simulink library "mantaFSHiLvl_cl"  (R2020a)
settings: Solver=VariableStepAuto  StartTime=0.0  StopTime=10.0  RelTol=1e-3
undefined symbols (not defined in the file or in its folder): fltCtrl, HILVLCONTROLLER, hiLvlCtrl, initializeBussesFromBlock
libraries: simulink x5, vectorMagnitude_ul x3, stopwatch_ul x1, pathFollowingControllerManta_cl x1
settings Model: Creator=mcobb  LastModifiedBy=JohnJr
settings DataIOCC: ReturnWorkspaceOutputs=off
settings DebuggingCC: ArithmeticOperatorsInVariantConditions=warning
settings SFSimCC: CustomCodeUndefinedFunction=UseInterfaceOnly

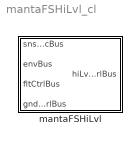
== system mantaFSHiLvl_cl ==
  mantaFSHiLvl : Subsystem  LoadFcn=initializeBussesFromBlock(gcb)  InitFcn=initializeBussesFromBlock(gcb)  StartFcn=initializeBussesFromBlock(gcb)  VariantControl=strcmpi(HILVLCONTROLLER,'mantaFSHiLvl')  mask{hiLvlCtrl=hiLvlCtrl}
      mask prompts: hiLvlCtrl "Hi-level controller"

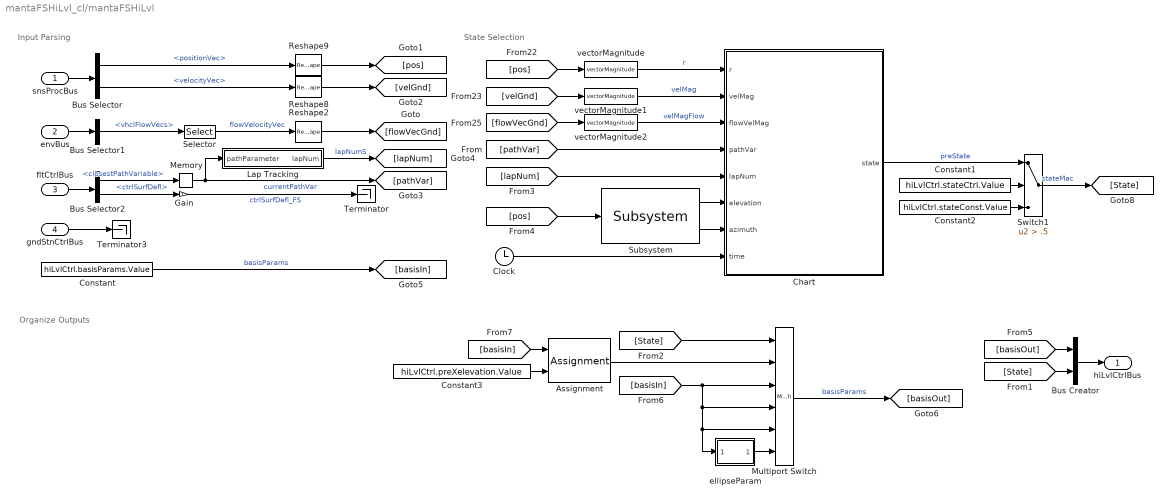
== system mantaFSHiLvl_cl/mantaFSHiLvl ==
  note: Organize Outputs
  note: Input Parsing
  note: State Selection
  snsProcBus : Inport  OutDataTypeStr=Bus: sensorsProcessingBus
  envBus : Inport  Port=2  OutDataTypeStr=Bus: envBus
  fltCtrlBus : Inport  Port=3  OutDataTypeStr=Bus: fltCtrlBus
  gndStnCtrlBus : Inport  Port=4  OutDataTypeStr=Bus: gndStnCtrlBus
  Assignment : Assignment  DiagnosticForDimensions=Warning  IndexOptions=Index vector (dialog)  Indices=3  OutputSizes=1
  Bus Creator : BusCreator  Inputs=2  OutDataTypeStr=Bus: hiLvlCtrlBus
  Bus Selector : BusSelector  OutputSignals=positionVec,velocityVec
  Bus Selector1 : BusSelector  OutputSignals=vhclFlowVecs
  Bus Selector2 : BusSelector  OutputSignals=closestPathVariable,ctrlSurfDefl
  Chart : Stateflow chart  TreatAsAtomicUnit=on  mask{nonXGain=fltCtrl.nonXCurrentSpoolInGain.Value, maxR=fltCtrl.maxTL.Value}
      mask prompts: nonXGain "non-xcurrent spool speed gain"; maxR "max kite position magnitude (r)"
  Clock : Clock
  Constant : Constant  Value=hiLvlCtrl.basisParams.Value
  Constant1 : Constant  Value=hiLvlCtrl.stateCtrl.Value
  Constant2 : Constant  Value=hiLvlCtrl.stateConst.Value
  Constant3 : Constant  Value=hiLvlCtrl.preXelevation.Value
  Gain : Gain
  Lap Tracking : Subsystem
  Memory : Memory
  Multiport Switch : MultiPortSwitch  Inputs=5
  Reshape2 : Reshape  OutputDimensionality=Column vector (2-D)
  Reshape8 : Reshape  OutputDimensionality=Column vector (2-D)
  Reshape9 : Reshape  OutputDimensionality=Column vector (2-D)
  Selector : Selector  NumberOfDimensions=2  InputPortWidth=3  IndexOptions=Select all,Index vector (dialog)  Indices=[1 3],5  OutputSizes=1,1
  Subsystem : pathFollowingControllerManta_cl/pathFollowingControllerManta/Subsystem  SystemSampleTime=-1  Latency=0  AutoFrameSizeCalculation=off
  Switch1 : Switch  Criteria=u2 > Threshold  Threshold=.5
  Terminator : Terminator
  Terminator3 : Terminator
  ellipseParam : Subsystem
  vectorMagnitude : vectorMagnitude_ul/vectorMagnitude  SystemSampleTime=-1  Latency=0  AutoFrameSizeCalculation=off
  vectorMagnitude1 : vectorMagnitude_ul/vectorMagnitude  SystemSampleTime=-1  Latency=0  AutoFrameSizeCalculation=off
  vectorMagnitude2 : vectorMagnitude_ul/vectorMagnitude  SystemSampleTime=-1  Latency=0  AutoFrameSizeCalculation=off
  hiLvlCtrlBus : Outport  OutDataTypeStr=Bus: hiLvlCtrlBus  VectorParamsAs1DForOutWhenUnconnected=off
  wires:
  gndStnCtrlBus/1 -> Terminator3/1
  Bus Creator/1 -> hiLvlCtrlBus/1
  Reshape9/1 -> [pos]
  snsProcBus/1 -> Bus Selector/1
  Reshape8/1 -> [velGnd]
  Bus Selector/2 -> Reshape8/1  "<velocityVec>"
  Bus Selector/1 -> Reshape9/1  "<positionVec>"
  Bus Selector1/1 -> Selector/1  "<vhclFlowVecs>"
  Reshape2/1 -> [flowVecGnd]
  envBus/1 -> Bus Selector1/1
  Selector/1 -> Reshape2/1  "flowVelocityVec"
  [State] -> Bus Creator/2
  [pos] -> vectorMagnitude/1
  [velGnd] -> vectorMagnitude1/1
  [flowVecGnd] -> vectorMagnitude2/1
  vectorMagnitude/1 -> Chart/1(r)  "r"
  vectorMagnitude1/1 -> Chart/2(velMag)  "velMag"
  vectorMagnitude2/1 -> Chart/3(flowVelMag)  "velMagFlow"
  fltCtrlBus/1 -> Bus Selector2/1
  Bus Selector2/1 -> Memory/1  "<closestPathVariable>"
  Memory/1 -> [pathVar], Lap Tracking/1(pathParameter)  "currentPathVar"
  Lap Tracking/1(lapNum) -> [lapNum]  "lapNumS"
  [pathVar] -> Chart/4(pathVar)
  [lapNum] -> Chart/5(lapNum)
  Subsystem/1 -> Chart/6(elevation)
  Subsystem/2 -> Chart/7(azimuth)
  [pos] -> Subsystem/1
  Clock/1 -> Chart/8(time)
  Switch1/1 -> [State]  "stateMac"
  Chart/1(state) -> Switch1/1  "preState"
  Constant1/1 -> Switch1/2
  Constant2/1 -> Switch1/3
  Constant/1 -> [basisIn]  "basisParams"
  [State] -> Multiport Switch/1
  [basisIn] -> Multiport Switch/3, Multiport Switch/4, Multiport Switch/5, ellipseParam/1(In1)
  ellipseParam/1(Out1) -> Multiport Switch/6
  Multiport Switch/1 -> [basisOut]  "basisParams"
  [basisOut] -> Bus Creator/1
  [basisIn] -> Assignment/1
  Assignment/1 -> Multiport Switch/2
  Constant3/1 -> Assignment/2
  Bus Selector2/2 -> Gain/1  "<ctrlSurfDefl>"
  Gain/1 -> Terminator/1  "ctrlSurfDefl_FS"

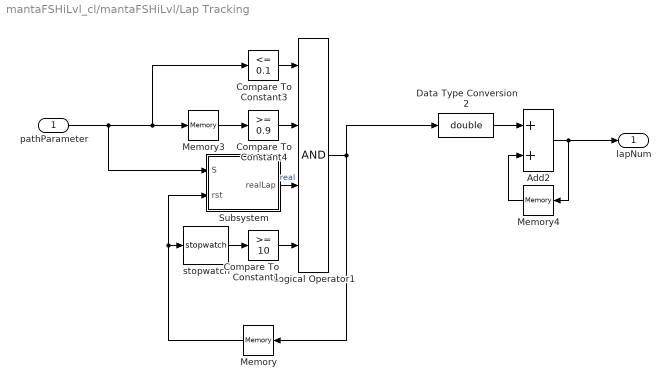
== system mantaFSHiLvl_cl/mantaFSHiLvl/Lap Tracking ==
  pathParameter : Inport
  Add2 : Sum
  Compare To Constant1 : simulink/Logic and Bit Operations/Compare To Constant  relop=>=  const=10  OutDataTypeStr=boolean
  Compare To Constant3 : simulink/Logic and Bit Operations/Compare To Constant  relop=<=  const=0.1  OutDataTypeStr=boolean
  Compare To Constant4 : simulink/Logic and Bit Operations/Compare To Constant  relop=>=  const=0.9  OutDataTypeStr=boolean
  Data Type Conversion2 : DataTypeConversion  OutDataTypeStr=double
  Logical Operator1 : Logic  Inputs=4  AllPortsSameDT=off  OutDataTypeStr=boolean
  Memory : Memory  InitialCondition=false
  Memory3 : Memory
  Memory4 : Memory
  Subsystem : Subsystem
  stopwatch : stopwatch_ul/stopwatch  SystemSampleTime=-1  Latency=0  AutoFrameSizeCalculation=off
  lapNum : Outport  VectorParamsAs1DForOutWhenUnconnected=off
  wires:
  Subsystem/1(realLap) -> Logical Operator1/3  "real"
  Compare To Constant1/1 -> Logical Operator1/4
  Memory/1 -> stopwatch/1, Subsystem/2(rst)
  stopwatch/1 -> Compare To Constant1/1
  pathParameter/1 -> Memory3/1, Compare To Constant3/1, Subsystem/1(S)
  Compare To Constant4/1 -> Logical Operator1/2
  Add2/1 -> Memory4/1, lapNum/1
  Memory4/1 -> Add2/2
  Logical Operator1/1 -> Memory/1, Data Type Conversion2/1
  Data Type Conversion2/1 -> Add2/1
  Memory3/1 -> Compare To Constant4/1
  Compare To Constant3/1 -> Logical Operator1/1

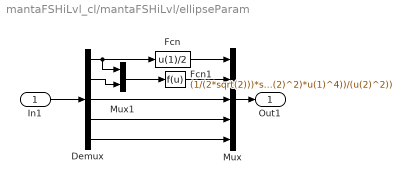
== system mantaFSHiLvl_cl/mantaFSHiLvl/ellipseParam ==
  In1 : Inport
  Demux : Demux  Outputs=5
  Fcn : Fcn  Expr=u(1)/2
  Fcn1 : Fcn  Expr=(1/(2*sqrt(2)))*sqrt(-u(1)^2+sqrt((u(2)^2*(4+u(2)^2)*u(1)^4))/(u(2)^2))
  Mux : Mux  Inputs=5
  Mux1 : Mux  Inputs=2
  Out1 : Outport
  wires:
  In1/1 -> Demux/1
  Mux1/1 -> Fcn1/1
  Demux/4 -> Mux/4
  Mux/1 -> Out1/1
  Fcn1/1 -> Mux/2
  Demux/2 -> Mux1/2
  Demux/1 -> Mux1/1, Fcn/1
  Fcn/1 -> Mux/1
  Demux/5 -> Mux/5
  Demux/3 -> Mux/3

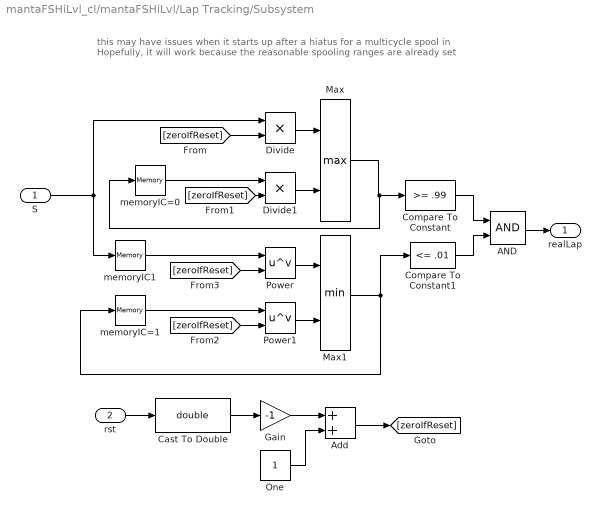
== system mantaFSHiLvl_cl/mantaFSHiLvl/Lap Tracking/Subsystem ==
  note: this may have issues when it starts up after a hiatus for a multicycle spool in
      | Hopefully, it will work because the reasonable spooling ranges are already set
  S : Inport
  rst : Inport  Port=2
  AND : Logic  AllPortsSameDT=off  OutDataTypeStr=boolean
  Add : Sum
  Cast To Double : DataTypeConversion  OutDataTypeStr=double
  Compare To Constant : simulink/Logic and Bit Operations/Compare To Constant  relop=>=  const=.99  OutDataTypeStr=boolean
  Compare To Constant1 : simulink/Logic and Bit Operations/Compare To Constant  relop=<=  const=.01  OutDataTypeStr=boolean
  Divide : Product  Inputs=**
  Divide1 : Product  Inputs=**
  Gain : Gain  Gain=-1
  Max : MinMax  Function=max  Inputs=2
  Max1 : MinMax  Inputs=2
  One : Constant  OutDataTypeStr=Inherit: Inherit via back propagation
  Power : Math  Operator=pow  SaturateOnIntegerOverflow=on
  Power1 : Math  Operator=pow  SaturateOnIntegerOverflow=on
  memoryIC1 : Memory  InitialCondition=1
  memoryIC=0 : Memory
  memoryIC=1 : Memory  InitialCondition=1
  realLap : Outport
  wires:
  memoryIC1/1 -> Power/1
  memoryIC=1/1 -> Power1/1
  [zeroIfReset] -> Power1/2
  memoryIC=0/1 -> Divide1/1
  Divide1/1 -> Max/2
  [zeroIfReset] -> Divide1/2
  [zeroIfReset] -> Power/2
  [zeroIfReset] -> Divide/2
  AND/1 -> realLap/1
  Compare To Constant1/1 -> AND/2
  Compare To Constant/1 -> AND/1
  Cast To Double/1 -> Gain/1
  Power1/1 -> Max1/2
  Power/1 -> Max1/1
  Max/1 -> Compare To Constant/1, memoryIC=0/1
  Divide/1 -> Max/1
  One/1 -> Add/2
  Add/1 -> [zeroIfReset]
  Gain/1 -> Add/1
  S/1 -> memoryIC1/1, Divide/1
  rst/1 -> Cast To Double/1
  Max1/1 -> memoryIC=1/1, Compare To Constant1/1

== stateflow chart mantaFSHiLvl_cl/mantaFSHiLvl/Chart ==
  state init
    state = 2;
  state non_x
    state = 1;
  state exit
    state = 4;
  state cross
    state = 3;
  (default) -> non_x
  non_x -> init : [and(velMag < 0.1 * flowVelMag * nonXGain,time > 1500)]
  init -> cross : [or(velMag > flowVelMag*.1,time>2500)]
  exit -> non_x : [velMag < flowVelMag]
  cross -> exit : [and(and(r > maxR, or(and(pathVar > .25, pathVar < .4),and(pathVar > .75,pathVar < .9))),lapNum >14)]
  data: r input; velMag input; flowVelMag input; nonXGain parameter; maxR parameter; pathVar input; lapNum input; state output =1; elevation input; azimuth input; time input
